simulink model "S12_Sound_Playground"  (R2026a)
settings: Solver=FixedStepDiscrete  StopTime=10  FixedStep=0.02
libraries: dspsnks4 x1
Description:
  | Synthetic Engine Sound Simulink Playground v0.9. Frozen physical/runtime cores are not modified.
settings Model: Creator=Jovi  LastModifiedBy=Jovi

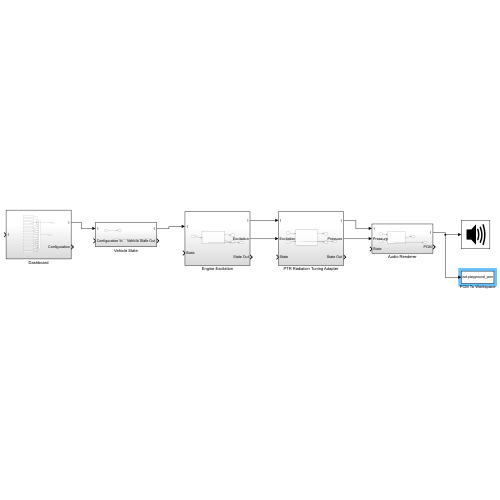
[thumbnail: Simulink's stored preview of the top-level diagram]
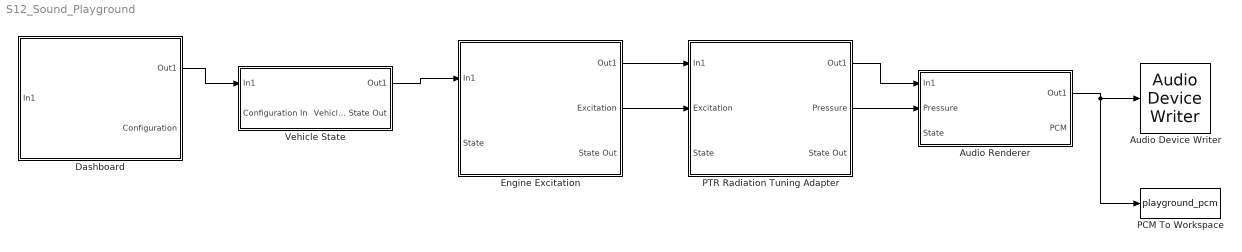
== system S12_Sound_Playground ==
  Audio Device Writer : dspsnks4/Audio Device Writer  Driver=DirectSound  Device=Default  InheritSampleRate=off  SampleRate=48000  BitDepth=24-bit integer  BufferSize=4096  NumBuffers=10  DefaultOutputChannelMapping=on  OutputChannelMapping=1:2  OutputNumUnderrunSamples=off  DriverIdx=1  DeviceWarnFlag=''
  Audio Renderer : Subsystem
  Dashboard : Subsystem
  Engine Excitation : Subsystem
  PCM To Workspace : ToWorkspace  VariableName=playground_pcm  SampleTime=-1
  PTR Radiation Tuning Adapter : Subsystem
  Vehicle State : Subsystem
  wires:
  Dashboard/1(Out1) -> Vehicle State/1(In1)
  Vehicle State/1(Out1) -> Engine Excitation/1(In1)
  Engine Excitation/1(Out1) -> PTR Radiation Tuning Adapter/1(In1)
  Engine Excitation/2(Excitation) -> PTR Radiation Tuning Adapter/2(Excitation)
  PTR Radiation Tuning Adapter/1(Out1) -> Audio Renderer/1(In1)
  PTR Radiation Tuning Adapter/2(Pressure) -> Audio Renderer/2(Pressure)
  Audio Renderer/1(Out1) -> Audio Device Writer/1, PCM To Workspace/1

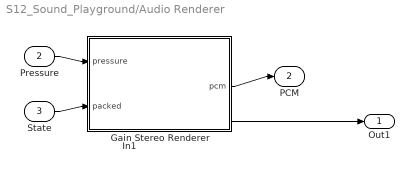
== system S12_Sound_Playground/Audio Renderer ==
  In1 : Inport
  Pressure : Inport  Port=2
  State : Inport  Port=3
  Gain Stereo Renderer : MATLAB Function  TreatAsAtomicUnit=on
  Out1 : Outport
  PCM : Outport  Port=2
  wires:
  In1/1 -> Out1/1
  Pressure/1 -> Gain Stereo Renderer/1(pressure)
  State/1 -> Gain Stereo Renderer/2(packed)
  Gain Stereo Renderer/1(pcm) -> PCM/1

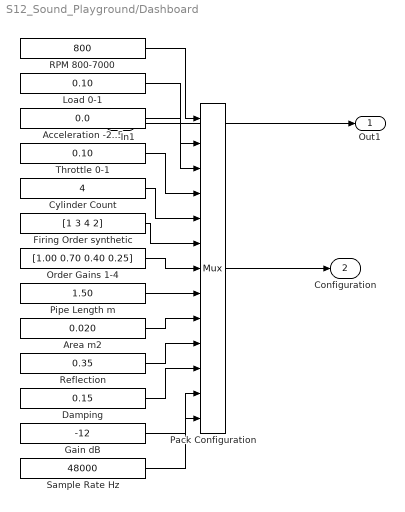
== system S12_Sound_Playground/Dashboard ==
  In1 : Inport
  Acceleration -2..5 : Constant  Value=0.0
  Area m2 : Constant  Value=0.020
  Cylinder Count : Constant  Value=4
  Damping : Constant  Value=0.15
  Firing Order synthetic : Constant  Value=[1 3 4 2]
  Gain dB : Constant  Value=-12
  Load 0-1 : Constant  Value=0.10
  Order Gains 1-4 : Constant  Value=[1.00 0.70 0.40 0.25]
  Pack Configuration : Mux  Inputs=13
  Pipe Length m : Constant  Value=1.50
  RPM 800-7000 : Constant  Value=800
  Reflection : Constant  Value=0.35
  Sample Rate Hz : Constant  Value=48000
  Throttle 0-1 : Constant  Value=0.10
  Out1 : Outport
  Configuration : Outport  Port=2
  wires:
  In1/1 -> Out1/1
  RPM 800-7000/1 -> Pack Configuration/1
  Load 0-1/1 -> Pack Configuration/2
  Acceleration -2..5/1 -> Pack Configuration/3
  Throttle 0-1/1 -> Pack Configuration/4
  Cylinder Count/1 -> Pack Configuration/5
  Firing Order synthetic/1 -> Pack Configuration/6
  Order Gains 1-4/1 -> Pack Configuration/7
  Pipe Length m/1 -> Pack Configuration/8
  Area m2/1 -> Pack Configuration/9
  Reflection/1 -> Pack Configuration/10
  Damping/1 -> Pack Configuration/11
  Gain dB/1 -> Pack Configuration/12
  Sample Rate Hz/1 -> Pack Configuration/13
  Pack Configuration/1 -> Configuration/1

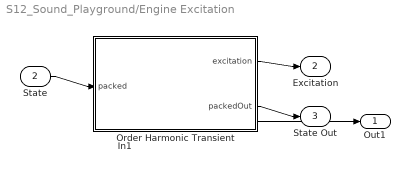
== system S12_Sound_Playground/Engine Excitation ==
  In1 : Inport
  State : Inport  Port=2
  Order Harmonic Transient : MATLAB Function  TreatAsAtomicUnit=on
  Out1 : Outport
  Excitation : Outport  Port=2
  State Out : Outport  Port=3
  wires:
  In1/1 -> Out1/1
  State/1 -> Order Harmonic Transient/1(packed)
  Order Harmonic Transient/1(excitation) -> Excitation/1
  Order Harmonic Transient/2(packedOut) -> State Out/1

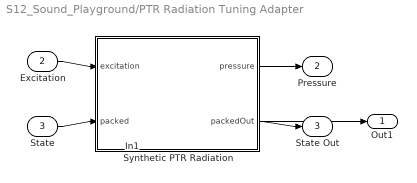
== system S12_Sound_Playground/PTR Radiation Tuning Adapter ==
  In1 : Inport
  Excitation : Inport  Port=2
  State : Inport  Port=3
  Synthetic PTR Radiation : MATLAB Function  TreatAsAtomicUnit=on
  Out1 : Outport
  Pressure : Outport  Port=2
  State Out : Outport  Port=3
  wires:
  In1/1 -> Out1/1
  Excitation/1 -> Synthetic PTR Radiation/1(excitation)
  State/1 -> Synthetic PTR Radiation/2(packed)
  Synthetic PTR Radiation/1(pressure) -> Pressure/1
  Synthetic PTR Radiation/2(packedOut) -> State Out/1

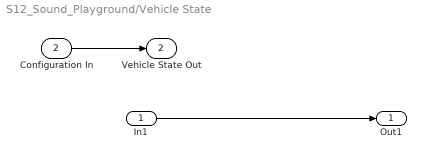
== system S12_Sound_Playground/Vehicle State ==
  In1 : Inport
  Configuration In : Inport  Port=2
  Out1 : Outport
  Vehicle State Out : Outport  Port=2
  wires:
  In1/1 -> Out1/1
  Configuration In/1 -> Vehicle State Out/1

== matlab function S12_Sound_Playground/Engine Excitation/Order Harmonic Transient ==
  data: packed input; excitation output; packedOut output
function [excitation, packedOut] = fcn(packed)
%#codegen
excitation = s12_sound_playground_excitation_step(packed(1), packed(2), packed(3), packed(4), packed(5), packed(6:9), packed(10:13), false);
packedOut = packed;
end

== matlab function S12_Sound_Playground/Audio Renderer/Gain Stereo Renderer ==
  data: pressure input; pcm output; packed input
function pcm = fcn(pressure, packed)
%#codegen
gain = 10^(packed(18) / 20);
pcm = gain * [pressure, pressure];
end

== matlab function S12_Sound_Playground/PTR Radiation Tuning Adapter/Synthetic PTR Radiation ==
  data: excitation input; pressure output; packed input; packedOut output
function [pressure, packedOut] = fcn(excitation, packed)
%#codegen
pressure = s12_sound_playground_ptr_tuning_step(excitation, packed(14), packed(15), packed(16), packed(17), false);
packedOut = packed;
end
